simulink model "step2"  (R2026a)
settings: Solver=VariableStepAuto
values from neighbouring files (symbols this model uses):
  Cd = Cd_values(k)    [cdstudy.m]
  m = masses(k)    [laptimestudy.m]
undefined symbols (not defined in the file or in its folder): A, F_drive, rho
settings Model: Creator=manoj  LastModifiedBy=manoj

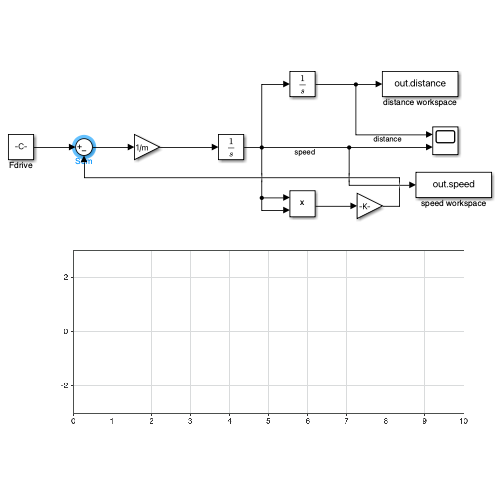
[thumbnail: Simulink's stored preview of the top-level diagram]
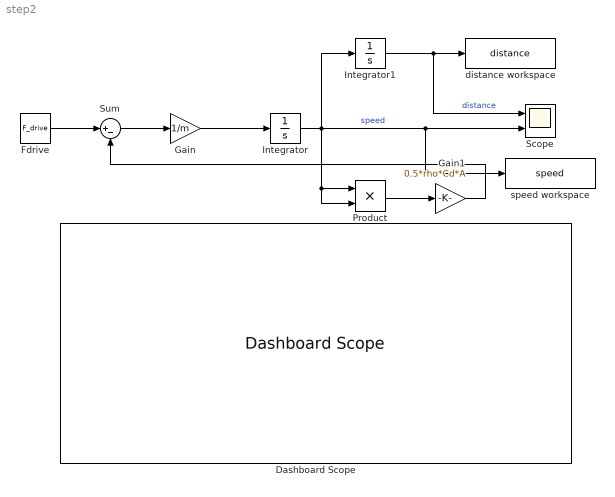
== system step2 ==
  Dashboard Scope : DashboardScope  FontColor=[0.0, 0.0, 0.0]
  Fdrive : Constant  Value=F_drive
  Gain : Gain  Gain=1/m
  Gain1 : Gain  Gain=0.5*rho*Cd*A
  Integrator : Integrator
  Integrator1 : Integrator
  Product : Product
  Scope : Scope  NumInputPorts=2
      settings: ActiveDisplayYMinimum=-1  ActiveDisplayYMaximum=1
  Sum : Sum  Inputs=|+-
  distance workspace : ToWorkspace  VariableName=distance  SaveFormat=Structure With Time  SampleTime=-1
  speed workspace : ToWorkspace  VariableName=speed  SaveFormat=Structure With Time  SampleTime=-1
  wires:
  Integrator/1 -> Product/2, Product/1, Integrator1/1, speed workspace/1, Scope/2  "speed"
  Gain/1 -> Integrator/1
  Gain1/1 -> Sum/2
  Product/1 -> Gain1/1
  Sum/1 -> Gain/1
  Fdrive/1 -> Sum/1
  Integrator1/1 -> distance workspace/1, Scope/1  "distance"
